simulink model "battery_dab_inv_single_phase"  (R2024b)
settings: Solver=ode1be  StartTime=0.0  StopTime=simlength  FixedStep=ts_sim  MaxStep=ts_sim
values from neighbouring files (symbols this model uses):
  Adrso = eye(2) + Arso*ts_dab    [init_model.m]
  Crso = [1 0]    [init_model.m]
  dead_time = 0    [init_model.m]
  DThs_init = 0    [init_model.m]
  freq = 50    [init_model.m]
  frequency_grid = 50    [init_model.m]
  I_FS = Iout_dc_nom * margin_factor    (= 37.5)    [init_model.m]
  Iout_dc_nom = 30    [init_model.m]
  ki_i_inv = 18    [init_model.m]
  ki_pll = 3140    [init_model.m]
  ki_v_inv = 12    [init_model.m]
  kp_i_inv = 0.5    [init_model.m]
  kp_pll = 314    [init_model.m]
  kp_v_inv = 0.2    [init_model.m]
  Ldrso = acker(Adrso',Crso',polesdrso)'    [init_model.m]
  number_of_cells = 30    [init_model.m]
  Q = 1000    [init_model.m]
  q1Kalman = ts_dab^2    (= 4e-08)    [init_model.m]
  q1kalman = 1    [init_model.m]
  q2Kalman = ts_dab^1    (= 0.0002)    [init_model.m]
  q2kalman = 1    [init_model.m]
  q3Kalman = 0    [init_model.m]
  rKalman = 1    [init_model.m]
  Rkalman = 1    [init_model.m]
  Tambient = 40    [init_model.m]
  tc = ts    (= 1e-06)    [init_model.m]
  V_FS = Vout_dc_nom * margin_factor    (= 500)    [init_model.m]
  Vout_dc_nom = 400    [init_model.m]
  w = 2*pi*f    (= 314.159265359)    [init_model.m]
  weigth = 0.6/6    (= 0.1)    [init_model.m]
undefined symbols (not defined in the file or in its folder): Aresd, Bresd, Cresd, fPWM_INV, fPWM_ZVS, ki_i_zvs, ki_v_zvs, kp_i_zvs, kp_v_zvs, magnitude, ts_inv, ts_zvs, tsample
libraries: fl_lib x136, nesl_utility x98, ee_lib x21, cstblocks x7, lithium_ion_cell_lib x1, simulink x1, single_phase_transformer_lib x1
(part 7 of 7)

== matlab function battery_dab_inv_single_phase/inverter_modA/single phase inverter control/dqbased_single_phase_inverter_ctrl/alpha_beta_transformation_u/kalman_observer ==
  data: y input; h1_hat output; w input; Ts input; q1 input; q2 input; r input; h2_hat output
function [h1_hat, h2_hat]   = KFO(y,w,Ts,q1,q2,r)

    persistent   x1_po x2_po p11_po p12_po p21_po p22_po

    if isempty(x1_po)
        x1_po = 0;
        x2_po = 0;
        p11_po = 0;
        p12_po = 0;
        p21_po = 0;
        p22_po = 0;        
    end
    
    a11 = cos(w*Ts);
    a12 = sin(w*Ts);
    a21 = -sin(w*Ts);
    a22 = cos(w*Ts);
    
    x1_pr = a11*x1_po + a12*x2_po;
    x2_pr = a21*x1_po + a22*x2_po;
    
    p11_pr = q1 + a11*(a11*p11_po+a12*p21_po) + a12*(a11*p12_po+a12*p22_po);
    p12_pr = a21*(a11*p11_po+a12*p21_po) + a22*(a11*p12_po+a12*p22_po);
    p21_pr = a11*(a21*p11_po+a22*p21_po) + a12*(a21*p12_po+a22*p22_po);
    p22_pr = q2 + a21*(a21*p11_po+a22*p21_po) + a22*(a21*p12_po+a22*p22_po);
    
    l1 = p11_pr/(p11_pr + r);
    l2 = p21_pr/(p11_pr + r);
    
    x1_po = x1_pr + l1*(y-x1_pr);
    x2_po = x2_pr + l2*(y-x1_pr);
    
    p11_po = (1-l1)*p11_pr;
    p12_po = (1-l1)*p12_pr;
    p21_po = p21_pr-l2*p11_pr;
    p22_po = p22_pr-l2*p12_pr;
    
    h1_hat = x1_pr;
    h2_hat = x2_pr;
end

== matlab function battery_dab_inv_single_phase/inverter_modA/single_phase_pll/xieta2alphabeta ==
  data: xi input; alpha output; eta input; gamma input; beta output
function [alpha,beta] = xieta2alphabeta(xi,eta,gamma)
    alpha  = xi*cos(gamma) - eta*sin(gamma);
    beta = xi*sin(gamma) + eta*cos(gamma);
end

== matlab function battery_dab_inv_single_phase/line_source/phase_gen/bounder1 ==
  data: u input; y output
function y = bounder(u)
    
    y = -pi + mod(u+3*pi,2*pi);
end

== matlab function battery_dab_inv_single_phase/inverter_modA/single phase inverter control/dqbased_single_phase_inverter_ctrl/flt_dq_d_i ==
  data: input input; y output
function y  = flt_dq_d(input)

FLTD2Q_B1 = 0.000966531084866133;
FLTD2Q_B2 = 0.000946498544476605;
FLTD2Q_A1 = -1.93814485260962;
FLTD2Q_A2 = 0.939101367424292;

    persistent x1 x2 y1 y2

    if isempty(x1)
        x1=0;
        x2=0;
        y1=0;
        y2=0;
    end


    o = x1 * FLTD2Q_B1 + x2 * FLTD2Q_B2 - y1 * FLTD2Q_A1 - y2 * FLTD2Q_A2;
    x2 = x1;
    x1 = input;
    y2 = y1;
    y1 = o;
	y = o;
end

== matlab function battery_dab_inv_single_phase/inverter_modA/single phase inverter control/dqbased_single_phase_inverter_ctrl/flt_dq_d_u ==
  data: input input; y output
function y  = flt_dq_d(input)

FLTD2Q_B1 = 0.000966531084866133;
FLTD2Q_B2 = 0.000946498544476605;
FLTD2Q_A1 = -1.93814485260962;
FLTD2Q_A2 = 0.939101367424292;

    persistent x1 x2 y1 y2

    if isempty(x1)
        x1=0;
        x2=0;
        y1=0;
        y2=0;
    end


    o = x1 * FLTD2Q_B1 + x2 * FLTD2Q_B2 - y1 * FLTD2Q_A1 - y2 * FLTD2Q_A2;
    x2 = x1;
    x1 = input;
    y2 = y1;
    y1 = o;
	y = o;
end

== matlab function battery_dab_inv_single_phase/dab_modA/battery_system/LithiumIonBattery/SOC_estimator/Kalman_observer/kalman_observer_gains ==
  data: i input; ts input; l1 output; z input; q1 input; q2 input; q3 input; r input; Q input; l2 output; l3 output
function [l1,l2,l3] = EKF(i,ts,z,q1,q2,q3,r,Q)

    persistent  p11 p12 p13 p21 p22 p23 p31 p32 p33

    if isempty(p11)
        p11 = q1;
        p12 = 0;
        p13 = 0;
        p21 = 0;
        p22 = q2;
        p23 = 0;
        p31 = 0;
        p32 = 0;
        p33 = q3;
    end
    R = 0.15;
    C = 10;
    M = 125;
    E_1 = -1.031;
    E1 = 0.2156;
    E2 = 0;
    E3 = 0;
    Elog = -0.05;
    alpha = 35;

    a11 = 1;
    a12 = 0;
    a13 = 0;
    a21 = 0;
    a22 = exp(-ts/(R*C));
    a23 = 0;
    a31 = 0;
    a32 = 0;
    a33 = abs(exp(-i*ts/Q));

    c1 = -alpha*E_1*abs(exp(-alpha*z)) + E1 + 2*E2*z + 3*E3*z^2 - Elog/(1-z+ts);
    c2 = -R;
    c3 = M;
    
    p11_pr = a11*(a11*p11 + a12*p21 + a13*p31) + a12*(a11*p12 + a12*p22 + a13*p32) + a13*(a11*p13 + a12*p23 + a13*p33) + q1;

    p12_pr = a21*(a11*p11 + a12*p21 + a13*p31) + a22*(a11*p12 + a12*p22 + a13*p32) + a23*(a11*p13 + a12*p23 + a13*p33);

    p13_pr = a31*(a11*p11 + a12*p21 + a13*p31) + a32*(a11*p12 + a12*p22 + a13*p32) + a33*(a11*p13 + a12*p23 + a13*p33);

    p21_pr = a11*(a21*p11 + a22*p21 + a23*p31) + a12*(a21*p12 + a22*p22 + a23*p32) + a13*(a21*p13 + a22*p23 + a23*p33);

    p22_pr = a21*(a21*p11 + a22*p21 + a23*p31) + a22*(a21*p12 + a22*p22 + a23*p32) + a23*(a21*p13 + a22*p23 + a23*p33) + q2;

    p23_pr = a31*(a21*p11 + a22*p21 + a23*p31) + a32*(a21*p12 + a22*p22 + a23*p32) + a33*(a21*p13 + a22*p23 + a23*p33);

    p31_pr = a11*(a31*p11 + a32*p21 + a33*p31) + a12*(a31*p12 + a32*p22 + a33*p32) + a13*(a31*p13 + a32*p23 + a33*p33);

    p32_pr = a21*(a31*p11 + a32*p21 + a33*p31) + a22*(a31*p12 + a32*p22 + a33*p32) + a23*(a31*p13 + a32*p23 + a33*p33);

    p33_pr = a31*(a31*p11 + a32*p21 + a33*p31) + a32*(a31*p12 + a32*p22 + a33*p32) + a33*(a31*p13 + a32*p23 + a33*p33) + q3;

    den = c1*(c1*p11 + c2*p21 + c3*p31) + c2*(c1*p12 + c2*p22 + c3*p32) + c3*(c1*p13 + c2*p23 + c3*p33) + r;
 
    l1 = (c1*p11 + c2*p12 + c3*p13)/den;
    l2 = (c1*p21 + c2*p22 + c3*p23)/den;
    l3 = (c1*p31 + c2*p32 + c3*p33)/den;
    
    p11 = (1 - c1*l1)*p11_pr - c2*l1*p21_pr - c3*l1*p31_pr;
    
    p12 = (1 - c1*l1)*p12_pr - c2*l1*p22_pr - c3*l1*p32_pr;
    
    p13 = (1 - c1*l1)*p13_pr - c2*l1*p23_pr - c3*l1*p33_pr;
    
    p21 = -c1*l2*p11_pr + (1 - c2*l2)*p21_pr - c3*l2*p31_pr;
    
    p22 = -c1*l2*p12_pr + (1 - c2*l2)*p22_pr - c3*l2*p32_pr;
    
    p23 = -c1*l2*p13_pr + (1 - c2*l2)*p23_pr - c3*l2*p33_pr;
    
    p31 = -c1*l3*p11_pr - c2*l3*p21_pr + (1 - c3*l3)*p31_pr;
    
    p32 = -c1*l3*p12_pr - c2*l3*p22_pr + (1 - c3*l3)*p32_pr;
    
    p33 = -c1*l3*p13_pr - c2*l3*p23_pr + (1 - c3*l3)*p33_pr;
end

== matlab function battery_dab_inv_single_phase/inverter_modA/single_phase_pll/alphabeta2xieta ==
  data: alpha input; xi output; beta input; gamma input; eta output
function [xi,eta] = alphabeta2xieta(alpha,beta,gamma)
    xi  =  alpha*cos(gamma) + beta*sin(gamma);
    eta = -alpha*sin(gamma) + beta*cos(gamma);
end

== matlab function battery_dab_inv_single_phase/dab_modA/battery_system/LithiumIonBattery/SOC_estimator/Kalman_observer/lithium-ion battery model ==
  data: i input; SOC output; u output; ts input; Q input; l1 input; l2 input; l3 input; vout input; x output
function [SOC, u, x] = lithium_ion_battery(i,ts,Q,l1,l2,l3,vout)

    persistent z_po ir_po h_po vout_hat

    if isempty(z_po)
        ir_po = 0;
        h_po = 0;
        z_po = 0.35;        
    end
    
        R0 = 0.15;
        R = 0.15;
        C = 0.1;
        M = 125;
        E_1 = -1.031;
        E0 = 3.685;
        E1 = 0.2156;
        E2 = 0;
        E3 = 0;
        Elog = -0.05;
        alpha = 35;
        N = 100;
        
        z_pr = z_po - ts/Q*i ;
    
        ir_pr = exp(-ts/(R*C))*ir_po + (1-exp(-ts/(R*C)))*i;

        h_pr = exp(-abs(i)*ts/Q)*h_po - (1-exp(-abs(i)*ts/Q))*sign(i);
        
        OCV = E_1*exp(-z_pr*alpha) + E0 + E1*z_pr + E2*z_pr^2 + E3*z_pr^3 + Elog*log(1-z_pr+ts);
        
        vout_hat = OCV*N + M*h_pr - R*ir_pr - R0*i;
        
        z_po = z_pr + l1*(vout - vout_hat);
        ir_po = ir_pr + l2*(vout - vout_hat);
        h_po = h_pr + l3*(vout - vout_hat);
        u = vout_hat;
        
        x = [z_po; ir_po; h_po];

    SOC = z_po;
end
